simulink model "continious_profusion"  (R2024b)
settings: Solver=VariableStepAuto  StartTime=0.0  StopTime=500  RelTol=1e-3
model workspace (MAT data in the model file):
  k = Simulink.Parameter
  k.Value = 0.015
  k.Complexity = 'real'
  k.Dimensions = [1 1]
  k.DataType = 'auto'
  k_e = 10
settings Model: Creator=sunzi  LastModifiedBy=sunzi

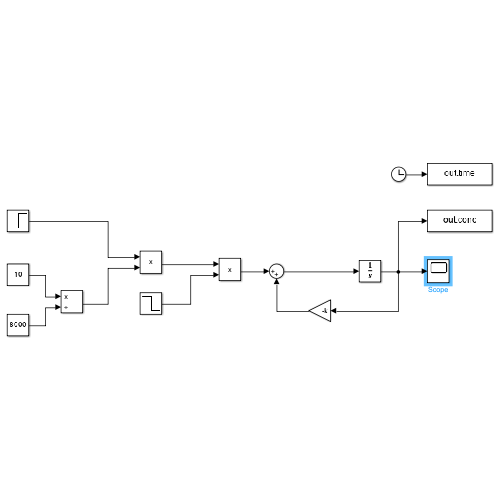
[thumbnail: Simulink's stored preview of the top-level diagram]
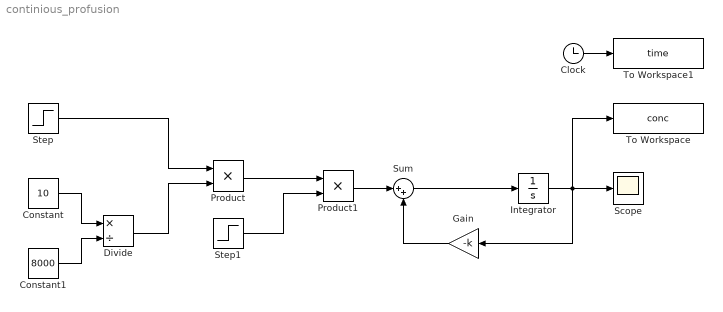
== system continious_profusion ==
  Clock : Clock
  Constant : Constant  Value=10
  Constant1 : Constant  Value=8000
  Divide : Product  Inputs=*/
  Gain : Gain  Gain=-k
  Integrator : Integrator
  Product : Product
  Product1 : Product
  Scope : Scope
  Step : Step  SampleTime=0
  Step1 : Step  Time=300  Before=1  After=0  SampleTime=0
  Sum : Sum  Inputs=|++
  To Workspace : ToWorkspace  VariableName=conc  SampleTime=-1
  To Workspace1 : ToWorkspace  VariableName=time  SaveFormat=Timeseries  SampleTime=-1
  wires:
  Step/1 -> Product/1
  Constant/1 -> Divide/1
  Constant1/1 -> Divide/2
  Divide/1 -> Product/2
  Product/1 -> Product1/1
  Sum/1 -> Integrator/1
  Integrator/1 -> To Workspace/1, Scope/1, Gain/1
  Gain/1 -> Sum/2
  Step1/1 -> Product1/2
  Product1/1 -> Sum/1
  Clock/1 -> To Workspace1/1
